simulink model "AutoManualManeuver"  (R2017b)
settings: Solver=FixedStepAuto  StartTime=0.0  StopTime=10.0  FixedStep=0.08  RelTol=1e-3
model workspace (MAT data in the model file):
  ContractValidatorBlocksMap = containers.Map
  ContractValidatorBlocksMap.serialization.keys = {'AutoManualManeuver/Logic/If AUTO/AUTO MANEUVER MODULE/req_s3_3_2_p27_1/validator', 'AutoManualManeuver/Logic/Req_s3_1_2_2_p19_5/validator', 'AutoManualManeuver/Logic/Req_s3_1_2_2_p19_5_part2/validator', 'AutoManualManeuver/Req_s3_1_2_2_p19_5_part1/validator', 'AutoManualManeuver/Req_s3_1_2_2_p19_5_part2/validator', 'AutoManualManeuver/contract/validator'}
  ContractValidatorBlocksMap.serialization.values{1}.block = 'AutoManualManeuver/Logic/If AUTO/AUTO MANEUVER MODULE/req_s3_3_2_p27_1/validator'
  ContractValidatorBlocksMap.serialization.values{1}.assumePorts = 1
  ContractValidatorBlocksMap.serialization.values{1}.guaranteePorts = 2
  ContractValidatorBlocksMap.serialization.values{1}.modeBlocksPorts = 0
  ContractValidatorBlocksMap.serialization.values{1}.portHandles.Inport = [4142.00036621 4143.00036621 4144.00036621]
  ContractValidatorBlocksMap.serialization.values{1}.portHandles.Outport = 4145.00036621
  ContractValidatorBlocksMap.serialization.values{1}.portHandles.Enable = []
  ContractValidatorBlocksMap.serialization.values{1}.portHandles.Trigger = []
  ContractValidatorBlocksMap.serialization.values{1}.portHandles.State = []
  ContractValidatorBlocksMap.serialization.values{1}.portHandles.LConn = []
  ContractValidatorBlocksMap.serialization.values{1}.portHandles.RConn = []
  ContractValidatorBlocksMap.serialization.values{1}.portHandles.Ifaction = []
  ContractValidatorBlocksMap.serialization.values{1}.portHandles.Reset = []
  ContractValidatorBlocksMap.serialization.values{1}.portConnectivity(1).Type = '1'
  ContractValidatorBlocksMap.serialization.values{1}.portConnectivity(1).Position = [365 -95]
  ContractValidatorBlocksMap.serialization.values{1}.portConnectivity(1).SrcBlock = 3623.00036621
  ContractValidatorBlocksMap.serialization.values{1}.portConnectivity(1).SrcPort = 0
  ContractValidatorBlocksMap.serialization.values{1}.portConnectivity(1).DstBlock = []
  ContractValidatorBlocksMap.serialization.values{1}.portConnectivity(1).DstPort = []
  ContractValidatorBlocksMap.serialization.values{1}.portConnectivity(2).Type = '2'
  ContractValidatorBlocksMap.serialization.values{1}.portConnectivity(2).Position = [365 75]
  ContractValidatorBlocksMap.serialization.values{1}.portConnectivity(2).SrcBlock = 3631.00061035
  ContractValidatorBlocksMap.serialization.values{1}.portConnectivity(2).SrcPort = 0
  ContractValidatorBlocksMap.serialization.values{1}.portConnectivity(2).DstBlock = []
  ContractValidatorBlocksMap.serialization.values{1}.portConnectivity(2).DstPort = []
  ContractValidatorBlocksMap.serialization.values{1}.portConnectivity(3).Type = '3'
  ContractValidatorBlocksMap.serialization.values{1}.portConnectivity(3).Position = [365 245]
  ContractValidatorBlocksMap.serialization.values{1}.portConnectivity(3).SrcBlock = 3645.00061035
  ContractValidatorBlocksMap.serialization.values{1}.portConnectivity(3).SrcPort = 0
  ContractValidatorBlocksMap.serialization.values{1}.portConnectivity(3).DstBlock = []
  ContractValidatorBlocksMap.serialization.values{1}.portConnectivity(3).DstPort = []
  ContractValidatorBlocksMap.serialization.values{1}.portConnectivity(4).Type = '1'
  ContractValidatorBlocksMap.serialization.values{1}.portConnectivity(4).Position = [500 75]
  ContractValidatorBlocksMap.serialization.values{1}.portConnectivity(4).SrcBlock = []
  ContractValidatorBlocksMap.serialization.values{1}.portConnectivity(4).SrcPort = []
  ContractValidatorBlocksMap.serialization.values{1}.portConnectivity(4).DstBlock = 3658.00036621
  ContractValidatorBlocksMap.serialization.values{1}.portConnectivity(4).DstPort = 0
  ContractValidatorBlocksMap.serialization.values{2}.block = 'AutoManualManeuver/Logic/Req_s3_1_2_2_p19_5/validator'
  ContractValidatorBlocksMap.serialization.values{2}.assumePorts = 0
  ContractValidatorBlocksMap.serialization.values{2}.guaranteePorts = 1
  ContractValidatorBlocksMap.serialization.values{2}.modeBlocksPorts = 0
  ContractValidatorBlocksMap.serialization.values{2}.portHandles.Inport = 9798.00244141
  ContractValidatorBlocksMap.serialization.values{2}.portHandles.Outport = 9719.00170898
  ContractValidatorBlocksMap.serialization.values{2}.portHandles.Enable = []
  ContractValidatorBlocksMap.serialization.values{2}.portHandles.Trigger = []
  ContractValidatorBlocksMap.serialization.values{2}.portHandles.State = []
  ContractValidatorBlocksMap.serialization.values{2}.portHandles.LConn = []
  ContractValidatorBlocksMap.serialization.values{2}.portHandles.RConn = []
  ContractValidatorBlocksMap.serialization.values{2}.portHandles.Ifaction = []
  ContractValidatorBlocksMap.serialization.values{2}.portHandles.Reset = []
  ContractValidatorBlocksMap.serialization.values{2}.portConnectivity(1).Type = '1'
  ContractValidatorBlocksMap.serialization.values{2}.portConnectivity(1).Position = [365 140]
  ContractValidatorBlocksMap.serialization.values{2}.portConnectivity(1).SrcBlock = 9639.00195312
  ContractValidatorBlocksMap.serialization.values{2}.portConnectivity(1).SrcPort = 0
  ContractValidatorBlocksMap.serialization.values{2}.portConnectivity(1).DstBlock = []
  ContractValidatorBlocksMap.serialization.values{2}.portConnectivity(1).DstPort = []
  ContractValidatorBlocksMap.serialization.values{2}.portConnectivity(2).Type = '1'
  ContractValidatorBlocksMap.serialization.values{2}.portConnectivity(2).Position = [515 140]
  ContractValidatorBlocksMap.serialization.values{2}.portConnectivity(2).SrcBlock = []
  ContractValidatorBlocksMap.serialization.values{2}.portConnectivity(2).SrcPort = []
  ContractValidatorBlocksMap.serialization.values{2}.portConnectivity(2).DstBlock = 9656.00195312
  ContractValidatorBlocksMap.serialization.values{2}.portConnectivity(2).DstPort = 0
  ContractValidatorBlocksMap.serialization.values{3}.block = 'AutoManualManeuver/Logic/Req_s3_1_2_2_p19_5_part2/validator'
  ContractValidatorBlocksMap.serialization.values{3}.assumePorts = 0
  ContractValidatorBlocksMap.serialization.values{3}.guaranteePorts = 1
  ContractValidatorBlocksMap.serialization.values{3}.modeBlocksPorts = 0
  ContractValidatorBlocksMap.serialization.values{3}.portHandles.Inport = 10004.0056152
  ContractValidatorBlocksMap.serialization.values{3}.portHandles.Outport = 10005.0059814
  ContractValidatorBlocksMap.serialization.values{3}.portHandles.Enable = []
  ContractValidatorBlocksMap.serialization.values{3}.portHandles.Trigger = []
  ContractValidatorBlocksMap.serialization.values{3}.portHandles.State = []
  ContractValidatorBlocksMap.serialization.values{3}.portHandles.LConn = []
  ContractValidatorBlocksMap.serialization.values{3}.portHandles.RConn = []
  ContractValidatorBlocksMap.serialization.values{3}.portHandles.Ifaction = []
  ContractValidatorBlocksMap.serialization.values{3}.portHandles.Reset = []
  ContractValidatorBlocksMap.serialization.values{3}.portConnectivity(1).Type = '1'
  ContractValidatorBlocksMap.serialization.values{3}.portConnectivity(1).Position = [360 140]
  ContractValidatorBlocksMap.serialization.values{3}.portConnectivity(1).SrcBlock = 8693.01147461
  ContractValidatorBlocksMap.serialization.values{3}.portConnectivity(1).SrcPort = 0
  ContractValidatorBlocksMap.serialization.values{3}.portConnectivity(1).DstBlock = []
  ContractValidatorBlocksMap.serialization.values{3}.portConnectivity(1).DstPort = []
  ContractValidatorBlocksMap.serialization.values{3}.portConnectivity(2).Type = '1'
  ContractValidatorBlocksMap.serialization.values{3}.portConnectivity(2).Position = [515 140]
  ContractValidatorBlocksMap.serialization.values{3}.portConnectivity(2).SrcBlock = []
  ContractValidatorBlocksMap.serialization.values{3}.portConnectivity(2).SrcPort = []
  ContractValidatorBlocksMap.serialization.values{3}.portConnectivity(2).DstBlock = 8698.01123047
  ContractValidatorBlocksMap.serialization.values{3}.portConnectivity(2).DstPort = 0
  ContractValidatorBlocksMap.serialization.values{4}.block = 'AutoManualManeuver/Req_s3_1_2_2_p19_5_part1/validator'
  ContractValidatorBlocksMap.serialization.values{4}.assumePorts = 0
  ContractValidatorBlocksMap.serialization.values{4}.guaranteePorts = 3
  ContractValidatorBlocksMap.serialization.values{4}.modeBlocksPorts = 0
  ContractValidatorBlocksMap.serialization.values{4}.portHandles.Inport = [4138.00061035 4139.00036621 4140.00036621]
  ContractValidatorBlocksMap.serialization.values{4}.portHandles.Outport = 4141.00036621
  ContractValidatorBlocksMap.serialization.values{4}.portHandles.Enable = []
  ContractValidatorBlocksMap.serialization.values{4}.portHandles.Trigger = []
  ContractValidatorBlocksMap.serialization.values{4}.portHandles.State = []
  ContractValidatorBlocksMap.serialization.values{4}.portHandles.LConn = []
  ContractValidatorBlocksMap.serialization.values{4}.portHandles.RConn = []
  ContractValidatorBlocksMap.serialization.values{4}.portHandles.Ifaction = []
  ContractValidatorBlocksMap.serialization.values{4}.portHandles.Reset = []
  ContractValidatorBlocksMap.serialization.values{4}.portConnectivity(1).Type = '1'
  ContractValidatorBlocksMap.serialization.values{4}.portConnectivity(1).Position = [370 -130]
  ContractValidatorBlocksMap.serialization.values{4}.portConnectivity(1).SrcBlock = 4059.00036621
  ContractValidatorBlocksMap.serialization.values{4}.portConnectivity(1).SrcPort = 0
  ContractValidatorBlocksMap.serialization.values{4}.portConnectivity(1).DstBlock = []
  ContractValidatorBlocksMap.serialization.values{4}.portConnectivity(1).DstPort = []
  ContractValidatorBlocksMap.serialization.values{4}.portConnectivity(2).Type = '2'
  ContractValidatorBlocksMap.serialization.values{4}.portConnectivity(2).Position = [370 40]
  ContractValidatorBlocksMap.serialization.values{4}.portConnectivity(2).SrcBlock = 4063.00061035
  ContractValidatorBlocksMap.serialization.values{4}.portConnectivity(2).SrcPort = 0
  ContractValidatorBlocksMap.serialization.values{4}.portConnectivity(2).DstBlock = []
  ContractValidatorBlocksMap.serialization.values{4}.portConnectivity(2).DstPort = []
  ContractValidatorBlocksMap.serialization.values{4}.portConnectivity(3).Type = '3'
  ContractValidatorBlocksMap.serialization.values{4}.portConnectivity(3).Position = [370 210]
  ContractValidatorBlocksMap.serialization.values{4}.portConnectivity(3).SrcBlock = 4067.00061035
  ContractValidatorBlocksMap.serialization.values{4}.portConnectivity(3).SrcPort = 0
  ContractValidatorBlocksMap.serialization.values{4}.portConnectivity(3).DstBlock = []
  ContractValidatorBlocksMap.serialization.values{4}.portConnectivity(3).DstPort = []
  ContractValidatorBlocksMap.serialization.values{4}.portConnectivity(4).Type = '1'
  ContractValidatorBlocksMap.serialization.values{4}.portConnectivity(4).Position = [520 40]
  ContractValidatorBlocksMap.serialization.values{4}.portConnectivity(4).SrcBlock = []
  ContractValidatorBlocksMap.serialization.values{4}.portConnectivity(4).SrcPort = []
  ContractValidatorBlocksMap.serialization.values{4}.portConnectivity(4).DstBlock = 4072.00036621
  ContractValidatorBlocksMap.serialization.values{4}.portConnectivity(4).DstPort = 0
  ContractValidatorBlocksMap.serialization.values{5}.block = 'AutoManualManeuver/Req_s3_1_2_2_p19_5_part2/validator'
  ContractValidatorBlocksMap.serialization.values{5}.assumePorts = 0
  ContractValidatorBlocksMap.serialization.values{5}.guaranteePorts = 1
  ContractValidatorBlocksMap.serialization.values{5}.modeBlocksPorts = 0
  ContractValidatorBlocksMap.serialization.values{5}.portHandles.Inport = 27036.0012207
  ContractValidatorBlocksMap.serialization.values{5}.portHandles.Outport = 27037.0009766
  ContractValidatorBlocksMap.serialization.values{5}.portHandles.Enable = []
  ContractValidatorBlocksMap.serialization.values{5}.portHandles.Trigger = []
  ContractValidatorBlocksMap.serialization.values{5}.portHandles.State = []
  ContractValidatorBlocksMap.serialization.values{5}.portHandles.LConn = []
  ContractValidatorBlocksMap.serialization.values{5}.portHandles.RConn = []
  ContractValidatorBlocksMap.serialization.values{5}.portHandles.Ifaction = []
  ContractValidatorBlocksMap.serialization.values{5}.portHandles.Reset = []
  ContractValidatorBlocksMap.serialization.values{5}.portConnectivity(1).Type = '1'
  ContractValidatorBlocksMap.serialization.values{5}.portConnectivity(1).Position = [360 140]
  ContractValidatorBlocksMap.serialization.values{5}.portConnectivity(1).SrcBlock = 26634.0003662
  ContractValidatorBlocksMap.serialization.values{5}.portConnectivity(1).SrcPort = 0
  ContractValidatorBlocksMap.serialization.values{5}.portConnectivity(1).DstBlock = []
  ContractValidatorBlocksMap.serialization.values{5}.portConnectivity(1).DstPort = []
  ContractValidatorBlocksMap.serialization.values{5}.portConnectivity(2).Type = '1'
  ContractValidatorBlocksMap.serialization.values{5}.portConnectivity(2).Position = [515 140]
  ContractValidatorBlocksMap.serialization.values{5}.portConnectivity(2).SrcBlock = []
  ContractValidatorBlocksMap.serialization.values{5}.portConnectivity(2).SrcPort = []
  ContractValidatorBlocksMap.serialization.values{5}.portConnectivity(2).DstBlock = 26639.0006104
  ContractValidatorBlocksMap.serialization.values{5}.portConnectivity(2).DstPort = 0
  ContractValidatorBlocksMap.serialization.values{6}.block = 'AutoManualManeuver/contract/validator'
  ContractValidatorBlocksMap.serialization.values{6}.assumePorts = 0
  ContractValidatorBlocksMap.serialization.values{6}.guaranteePorts = 4
  ContractValidatorBlocksMap.serialization.values{6}.modeBlocksPorts = 0
  ContractValidatorBlocksMap.serialization.values{6}.portHandles.Inport = [8429.00061035 8433.00061035 8430.00061035 8428.00061035]
  ContractValidatorBlocksMap.serialization.values{6}.portHandles.Outport = 8423.00085449
  ContractValidatorBlocksMap.serialization.values{6}.portHandles.Enable = []
  ContractValidatorBlocksMap.serialization.values{6}.portHandles.Trigger = []
  ContractValidatorBlocksMap.serialization.values{6}.portHandles.State = []
  ContractValidatorBlocksMap.serialization.values{6}.portHandles.LConn = []
  ContractValidatorBlocksMap.serialization.values{6}.portHandles.RConn = []
  ContractValidatorBlocksMap.serialization.values{6}.portHandles.Ifaction = []
  ContractValidatorBlocksMap.serialization.values{6}.portHandles.Reset = []
  ContractValidatorBlocksMap.serialization.values{6}.portConnectivity(1).Type = '1'
  ContractValidatorBlocksMap.serialization.values{6}.portConnectivity(1).Position = [365 -110]
  ContractValidatorBlocksMap.serialization.values{6}.portConnectivity(1).SrcBlock = -1
  ContractValidatorBlocksMap.serialization.values{6}.portConnectivity(1).SrcPort = []
  ContractValidatorBlocksMap.serialization.values{6}.portConnectivity(1).DstBlock = []
  ContractValidatorBlocksMap.serialization.values{6}.portConnectivity(1).DstPort = []
  ContractValidatorBlocksMap.serialization.values{6}.portConnectivity(2).Type = '2'
  ContractValidatorBlocksMap.serialization.values{6}.portConnectivity(2).Position = [365 15]
  ContractValidatorBlocksMap.serialization.values{6}.portConnectivity(2).SrcBlock = 9285.00170898
  ContractValidatorBlocksMap.serialization.values{6}.portConnectivity(2).SrcPort = 0
  ContractValidatorBlocksMap.serialization.values{6}.portConnectivity(2).DstBlock = []
  ContractValidatorBlocksMap.serialization.values{6}.portConnectivity(2).DstPort = []
  ContractValidatorBlocksMap.serialization.values{6}.portConnectivity(3).Type = '3'
  ContractValidatorBlocksMap.serialization.values{6}.portConnectivity(3).Position = [365 140]
  ContractValidatorBlocksMap.serialization.values{6}.portConnectivity(3).SrcBlock = -1
  ContractValidatorBlocksMap.serialization.values{6}.portConnectivity(3).SrcPort = []
  ContractValidatorBlocksMap.serialization.values{6}.portConnectivity(3).DstBlock = []
  ContractValidatorBlocksMap.serialization.values{6}.portConnectivity(3).DstPort = []
  ContractValidatorBlocksMap.serialization.values{6}.portConnectivity(4).Type = '4'
  ContractValidatorBlocksMap.serialization.values{6}.portConnectivity(4).Position = [365 265]
  ContractValidatorBlocksMap.serialization.values{6}.portConnectivity(4).SrcBlock = -1
  ContractValidatorBlocksMap.serialization.values{6}.portConnectivity(4).SrcPort = []
  ContractValidatorBlocksMap.serialization.values{6}.portConnectivity(4).DstBlock = []
  ContractValidatorBlocksMap.serialization.values{6}.portConnectivity(4).DstPort = []
  ContractValidatorBlocksMap.serialization.values{6}.portConnectivity(5).Type = '1'
  ContractValidatorBlocksMap.serialization.values{6}.portConnectivity(5).Position = [500 80]
  ContractValidatorBlocksMap.serialization.values{6}.portConnectivity(5).SrcBlock = []
  ContractValidatorBlocksMap.serialization.values{6}.portConnectivity(5).SrcPort = []
  ContractValidatorBlocksMap.serialization.values{6}.portConnectivity(5).DstBlock = 8346.00061035
  ContractValidatorBlocksMap.serialization.values{6}.portConnectivity(5).DstPort = 0
  ContractValidatorBlocksMap.serialization.uniformity = 0
  ContractValidatorBlocksMap.serialization.keyType = 'char'
  ContractValidatorBlocksMap.serialization.valueType = 'any'
undefined symbols (not defined in the file or in its folder): contractAfterSimulation, ContractAssumeBlock, contractBeforeSimulation, ContractBlock, ContractGuaranteeBlock, ContractValidatorBlock, saveValidatorParameters
libraries: MATLAB_Function_lib x7, sldvlib x5, simulink x1
settings Model: Creator=hbourbou  LastModifiedBy=hbourbou

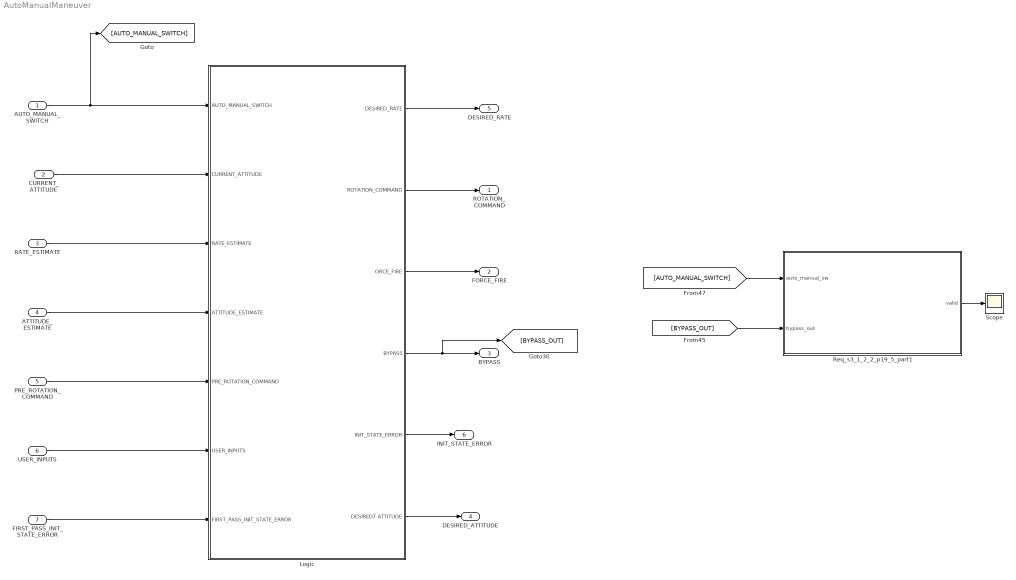
== system AutoManualManeuver ==
  AUTO_MANUAL_SWITCH : Inport  OutDataTypeStr=boolean  PortDimensions=1
  CURRENT_ATTITUDE : Inport  Port=2
  RATE_ESTIMATE : Inport  Port=3
  ATTITUDE_ESTIMATE : Inport  Port=4  PortDimensions=3
  PRE_ROTATION_COMMAND : Inport  Port=5  OutDataTypeStr=double  PortDimensions=3
  USER_INPUTS : Inport  Port=6  OutDataTypeStr=Bus: user_inputsBus
  FIRST_PASS_INIT_STATE_ERROR : Inport  Port=7
  Logic : Subsystem
  Req_s3_1_2_2_p19_5_part1 : Subsystem  mask(ContractBlock){ContractBlockType=ContractBlock}
      mask init:
      | set_param(gcb, 'LinkStatus', 'none');
      settings: CopyFcn=set_param(gcb, 'LinkStatus', 'none');
      mask DialogControl DescTextVar Prompt: Contract block
      mask Display:
      | text(0.5, 0.5, '{\bf\fontsize{20}Contract}', 'hor', 'center', 'texmode','on');
      | blocks = find_system(gcb, 'LookUnderMasks','all', 'SearchDepth',1,'BlockType','Inport');
      | for i = 1 : length(blocks)
      |     blockName = get_param(blocks(i), 'Name');
      |     [path, blockName] = fileparts(char(blockName));
      |     port_label('input', i, blockName);
      | end
      | 
      | blocks = find_system(gcb, 'LookUnderMasks','all', 'SearchDepth',1,'BlockType','Outport');
      | for i = 1 : length(blocks)
      |     blockName = get_param(blocks(i), 'Name');
      |     [path, blockName] = fileparts(char(blockName));
      |     port_label('output', i, blockName);
      | end
  Scope : Scope
  ROTATION_COMMAND : Outport  OutDataTypeStr=double  PortDimensions=3
  FORCE_FIRE : Outport  Port=2
  BYPASS : Outport  Port=3
  DESIRED_ATTITUDE : Outport  Port=4
  DESIRED_RATE : Outport  Port=5  OutDataTypeStr=double
  INIT_STATE_ERROR : Outport  Port=6
  wires:
  [AUTO_MANUAL_SWITCH] -> Req_s3_1_2_2_p19_5_part1/1(auto_manual_sw)
  [BYPASS_OUT] -> Req_s3_1_2_2_p19_5_part1/2(bypass_out)
  Req_s3_1_2_2_p19_5_part1/1(valid) -> Scope/1
  Logic/4(BYPASS) -> [BYPASS_OUT], BYPASS/1
  AUTO_MANUAL_SWITCH/1 -> [AUTO_MANUAL_SWITCH], Logic/1(AUTO_MANUAL_SWITCH)
  CURRENT_ATTITUDE/1 -> Logic/2(CURRENT_ATTITUDE)
  RATE_ESTIMATE/1 -> Logic/3(RATE_ESTIMATE)
  ATTITUDE_ESTIMATE/1 -> Logic/4(ATTITUDE_ESTIMATE)
  PRE_ROTATION_COMMAND/1 -> Logic/5(PRE_ROTATION_COMMAND)
  Logic/1(DESIRED_RATE) -> DESIRED_RATE/1
  Logic/2(ROTATION_COMMAND) -> ROTATION_COMMAND/1
  Logic/3(ORCE_FIRE) -> FORCE_FIRE/1
  USER_INPUTS/1 -> Logic/6(USER_INPUTS)
  FIRST_PASS_INIT_STATE_ERROR/1 -> Logic/7(FIRST_PASS_INIT_STATE_ERROR)
  Logic/6(DESIREDT ATTITUDE) -> DESIRED_ATTITUDE/1
  Logic/5(INIT_STATE_ERROR) -> INIT_STATE_ERROR/1

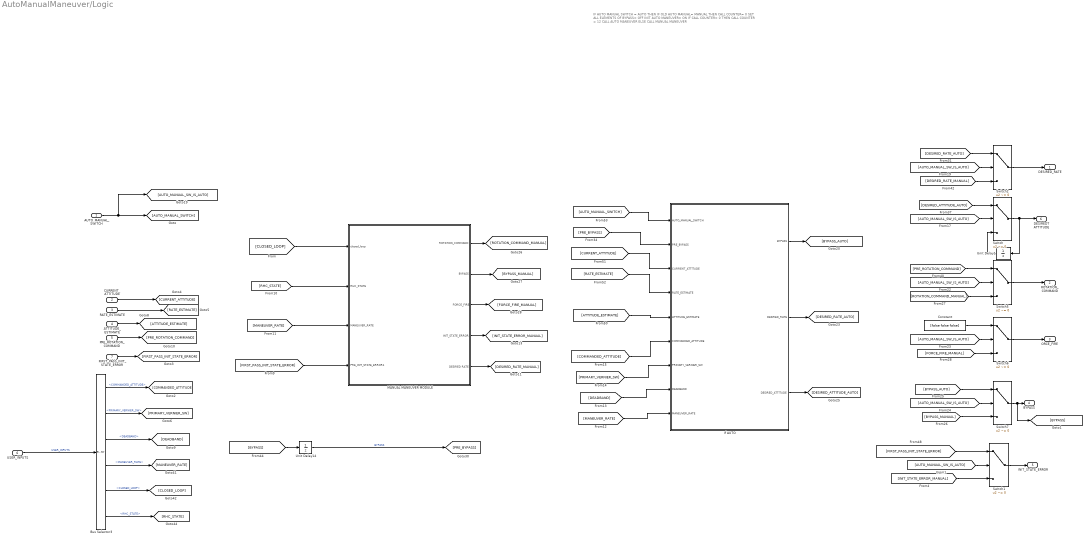
== system AutoManualManeuver/Logic ==
  note: IF AUTO MANUAL SWITCH = AUTO THEN
      | IF OLD AUTO MANUAL= MANUAL THEN
      | CALL COUNTER= 0
      | SET ALL ELEMENTS OF BYPASS= OFF
      | INIT AUTO MANEUVER= ON
      | IF CALL COUNTER= 0 THEN
      | CALL COUNTER = 12
      | CALL AUTO MANEUVER
      | ELSE CALL MANUAL MANEUVER
  AUTO_MANUAL_SWITCH : Inport
  CURRENT_ATTITUDE : Inport  Port=2
  RATE_ESTIMATE : Inport  Port=3
  ATTITUDE_ESTIMATE : Inport  Port=4
  PRE_ROTATION_COMMAND : Inport  Port=5
  USER_INPUTS : Inport  Port=6
  FIRST_PASS_INIT_STATE_ERROR : Inport  Port=7
  Bus Selector3 : BusSelector  OutputSignals=COMMANDED_ATTITUDE,PRIMARY_VERNIER_SW,DEADBAND,MANEUVER_RATE,CLOSED_LOOP,RHC_STATE
  Constant : Constant  Value=[false false false]
  If AUTO : Subsystem  TreatAsAtomicUnit=on
  MANUAL MANEUVER MODULE : Subsystem
  Switch{,1..2,5..7} (6 alike) : Switch  Criteria=u2 ~= 0
  Unit Delay1 : UnitDelay  InitialCondition=[0;0;0]  SampleTime=-1
  Unit Delay14 : UnitDelay  InitialCondition=[true; true; true]  SampleTime=-1
  DESIRED_RATE : Outport  OutDataTypeStr=double
  ROTATION_COMMAND : Outport  Port=2
  ORCE_FIRE : Outport  Port=3
  BYPASS : Outport  Port=4
  INIT_STATE_ERROR : Outport  Port=5
  DESIREDT ATTITUDE : Outport  Port=6  OutDataTypeStr=double
  wires:
  [RHC_STATE] -> MANUAL MANEUVER MODULE/2(RHC_STATE)
  [FIRST_PASS_INIT_STATE_ERROR] -> MANUAL MANEUVER MODULE/4(PRE_INIT_STATE_ERROR1)
  If AUTO/1(BYPASS) -> [BYPASS_AUTO]
  [CLOSED_LOOP] -> MANUAL MANEUVER MODULE/1(closed_loop)
  AUTO_MANUAL_SWITCH/1 -> [AUTO_MANUAL_SWITCH], [AUTO_MANUAL_SW_IS_AUTO]
  PRE_ROTATION_COMMAND/1 -> [PRE_ROTATION_COMMAND]
  [PRE_BYPASS] -> If AUTO/2(PRE_BYPASS)
  [AUTO_MANUAL_SWITCH] -> If AUTO/1(AUTO_MANUAL_SWITCH)
  [CURRENT_ATTITUDE] -> If AUTO/3(CURRENT_ATTITUDE)
  RATE_ESTIMATE/1 -> [RATE_ESTIMATE]
  ATTITUDE_ESTIMATE/1 -> [ATTITUDE_ESTIMATE]
  [RATE_ESTIMATE] -> If AUTO/4(RATE_ESTIMATE)
  CURRENT_ATTITUDE/1 -> [CURRENT_ATTITUDE]
  [ATTITUDE_ESTIMATE] -> If AUTO/5(ATTITUDE_ESTIMATE)
  Switch2/1 -> DESIRED_RATE/1
  Switch7/1 -> [BYPASS], BYPASS/1
  Switch5/1 -> ROTATION_COMMAND/1
  [MANEUVER_RATE] -> If AUTO/9(MANEUVER_RATE)
  [MANEUVER_RATE] -> MANUAL MANEUVER MODULE/3(MANEUVER_RATE)
  [COMMANDED_ATTITUDE] -> If AUTO/6(COMMANDED_ATTITUDE)
  Constant/1 -> Switch6/1
  [DEADBAND] -> If AUTO/8(DEADBAND)
  [PRE_ROTATION_COMMAND] -> Switch5/1
  [PRIMARY_VERNIER_SW] -> If AUTO/7(PRIMARY_VERNIER_SW)
  If AUTO/2(DESIRED_RATE) -> [DESIRED_RATE_AUTO]
  MANUAL MANEUVER MODULE/1(ROTATION_COMMAND) -> [ROTATION_COMMAND_MANUAL]
  MANUAL MANEUVER MODULE/2(BYPASS) -> [BYPASS_MANUAL]
  [DESIRED_RATE_MANUAL] -> Switch2/3
  [AUTO_MANUAL_SW_IS_AUTO] -> Switch2/2
  [DESIRED_RATE_AUTO] -> Switch2/1
  [ROTATION_COMMAND_MANUAL] -> Switch5/3
  [AUTO_MANUAL_SW_IS_AUTO] -> Switch7/2
  [AUTO_MANUAL_SW_IS_AUTO] -> Switch6/2
  [DESIRED_ATTITUDE_AUTO] -> Switch/1
  [BYPASS_MANUAL] -> Switch7/3
  [AUTO_MANUAL_SW_IS_AUTO] -> Switch5/2
  [FORCE_FIRE_MANUAL] -> Switch6/3
  [AUTO_MANUAL_SW_IS_AUTO] -> Switch/2
  If AUTO/3(DESIRED_ATTITUDE) -> [DESIRED_ATTITUDE_AUTO]
  MANUAL MANEUVER MODULE/3(FORCE_FIRE) -> [FORCE_FIRE_MANUAL]
  [BYPASS_AUTO] -> Switch7/1
  [BYPASS] -> Unit Delay14/1
  Unit Delay14/1 -> [PRE_BYPASS]  "BYPASS"
  Switch6/1 -> ORCE_FIRE/1
  Bus Selector3/6 -> [RHC_STATE]  "<RHC_STATE>"
  Bus Selector3/2 -> [PRIMARY_VERNIER_SW]  "<PRIMARY_VERNIER_SW>"
  Bus Selector3/5 -> [CLOSED_LOOP]  "<CLOSED_LOOP>"
  Bus Selector3/1 -> [COMMANDED_ATTITUDE]  "<COMMANDED_ATTITUDE>"
  Bus Selector3/3 -> [DEADBAND]  "<DEADBAND>"
  Bus Selector3/4 -> [MANEUVER_RATE]  "<MANEUVER_RATE>"
  USER_INPUTS/1 -> Bus Selector3/1  "USER_INPUTS"
  FIRST_PASS_INIT_STATE_ERROR/1 -> [FIRST_PASS_INIT_STATE_ERROR]
  MANUAL MANEUVER MODULE/5(DESIRED RATE) -> [DESIRED_RATE_MANUAL]
  [INIT_STATE_ERROR_MANUAL] -> Switch1/3
  [AUTO_MANUAL_SW_IS_AUTO] -> Switch1/2
  [FIRST_PASS_INIT_STATE_ERROR] -> Switch1/1
  Switch1/1 -> INIT_STATE_ERROR/1
  MANUAL MANEUVER MODULE/4(INIT_STATE_ERROR) -> [INIT_STATE_ERROR_MANUAL]
  Switch/1 -> Unit Delay1/1, DESIREDT ATTITUDE/1
  Unit Delay1/1 -> Switch/3

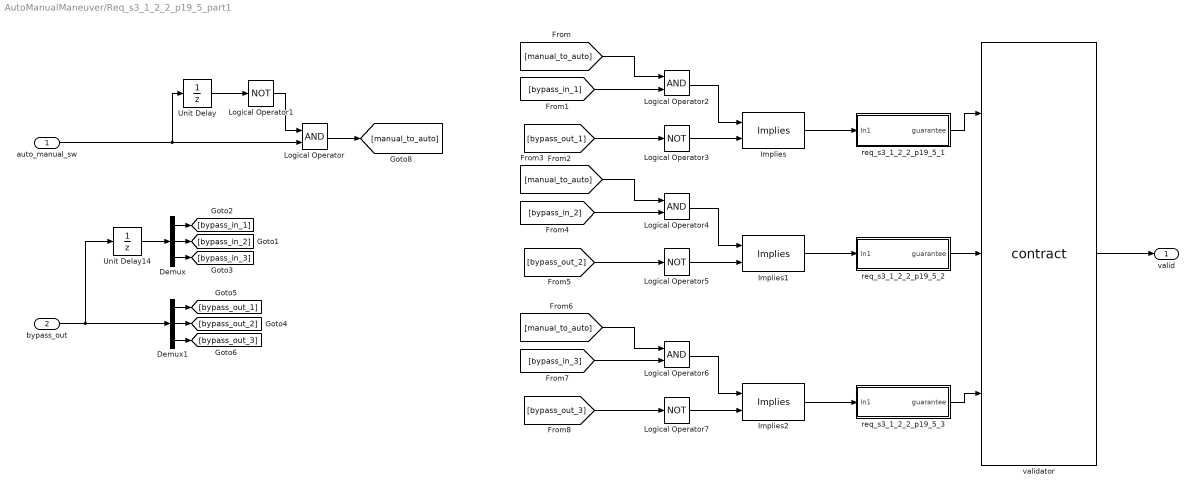
== system AutoManualManeuver/Req_s3_1_2_2_p19_5_part1 ==
  auto_manual_sw : Inport  OutDataTypeStr=boolean  PortDimensions=1
  bypass_out : Inport  Port=2
  Demux : Demux  Outputs=3
  Demux1 : Demux  Outputs=3
  Implies : sldvlib/Verification Utilities/Implies
      settings: SourceProductName=Simulink Design Verifier  SourceProductBaseCode=DV
  Implies1 : sldvlib/Verification Utilities/Implies
      settings: SourceProductName=Simulink Design Verifier  SourceProductBaseCode=DV
  Implies2 : sldvlib/Verification Utilities/Implies
      settings: SourceProductName=Simulink Design Verifier  SourceProductBaseCode=DV
  Logical Operator{,2,4,6} (4 alike) : Logic  AllPortsSameDT=off  OutDataTypeStr=boolean
  Logical Operator1 : Logic  Operator=NOT  Inputs=1  AllPortsSameDT=off  OutDataTypeStr=boolean
  Logical Operator3 : Logic  Operator=NOT  AllPortsSameDT=off  OutDataTypeStr=boolean
  Logical Operator5 : Logic  Operator=NOT  AllPortsSameDT=off  OutDataTypeStr=boolean
  Logical Operator7 : Logic  Operator=NOT  AllPortsSameDT=off  OutDataTypeStr=boolean
  Unit Delay : UnitDelay  InitialCondition=true  SampleTime=-1
  Unit Delay14 : UnitDelay  InitialCondition=[true; true; true]  SampleTime=-1
  req_s3_1_2_2_p19_5_1 : Subsystem  mask(ContractGuaranteeBlock){ContractBlockType=ContractGuaranteeBlock}
      mask init:
      | set_param(gcb, 'LinkStatus', 'none');
      mask DialogControl DescTextVar Prompt: Guarantee block
  req_s3_1_2_2_p19_5_2 : Subsystem  mask(ContractGuaranteeBlock){ContractBlockType=ContractGuaranteeBlock}
      mask init:
      | set_param(gcb, 'LinkStatus', 'none');
      mask DialogControl DescTextVar Prompt: Guarantee block
  req_s3_1_2_2_p19_5_3 : Subsystem  mask(ContractGuaranteeBlock){ContractBlockType=ContractGuaranteeBlock}
      mask init:
      | set_param(gcb, 'LinkStatus', 'none');
      mask DialogControl DescTextVar Prompt: Guarantee block
  validator : M-S-Function  LoadFcn=saveValidatorParameters(gcb);  InitFcn=contractBeforeSimulation();  StopFcn=contractAfterSimulation();  FunctionName=contract  mask(ContractValidatorBlock){assumePorts=0, guaranteePorts=3, modePorts=0, ContractBlockType=ContractValidatorBlock, createInportsCheckbox=off}
      mask prompts: assumePorts "Assume ports     :"; guaranteePorts "Guarantee ports :"; modePorts "Mode ports        :"; createInportsCheckbox "Create inports and connect them automatically"
      mask init:
      | set_param(gcb,'LinkStatus','none');
      | contract_callback('inputs_callback',gcb);
      mask DialogControl DescTextVar Prompt: The validator block implements the following logic: <br> <br> <b>Sofar</b>(assume<sub>1</sub> <b>&#8743;</b> assume<sub>2</sub> <b>&#8743;</b> ... assume<sub>k</sub>) <b>&rarr;</b> (guarantee<sub>1</sub> <b>&#8743;</b> guarantee<sub>2</sub> <b>&#8743;</b> ... guarantee<sub>m</sub> <b>&#8743;</b>  mode<sub>1</sub> <b>&#8743;</b> mode<sub>2</sub> <b>&#8743;</b> ... <b>&#8743;</b> mode<sub>n</sub> )<br> where mode<sub>i</sub> = require<sub>i</sub> <b>&rarr;</b> ensure<sub>i</sub>
      mask Display:
      | color('black');
      | port_label('input',1,'guarantee');
      | port_label('input',2,'guarantee');
      | port_label('input',3,'guarantee');
      | port_label('output',1,'valid');
  valid : Outport
  wires:
  validator/1 -> valid/1
  req_s3_1_2_2_p19_5_3/1(guarantee) -> validator/3
  Implies/1 -> req_s3_1_2_2_p19_5_1/1(In1)
  [manual_to_auto] -> Logical Operator2/1
  Demux/3 -> [bypass_in_3]
  Implies2/1 -> req_s3_1_2_2_p19_5_3/1(In1)
  Logical Operator3/1 -> Implies/2
  [bypass_in_3] -> Logical Operator6/2
  Unit Delay/1 -> Logical Operator1/1
  Demux1/2 -> [bypass_out_2]
  Demux/1 -> [bypass_in_1]
  Logical Operator1/1 -> Logical Operator/1
  bypass_out/1 -> Unit Delay14/1, Demux1/1
  Demux/2 -> [bypass_in_2]
  [bypass_out_1] -> Logical Operator3/1
  [manual_to_auto] -> Logical Operator4/1
  Logical Operator7/1 -> Implies2/2
  Logical Operator2/1 -> Implies/1
  [bypass_out_2] -> Logical Operator5/1
  Implies1/1 -> req_s3_1_2_2_p19_5_2/1(In1)
  [bypass_out_3] -> Logical Operator7/1
  Logical Operator5/1 -> Implies1/2
  [bypass_in_1] -> Logical Operator2/2
  Logical Operator4/1 -> Implies1/1
  Demux1/1 -> [bypass_out_1]
  Unit Delay14/1 -> Demux/1
  [bypass_in_2] -> Logical Operator4/2
  auto_manual_sw/1 -> Logical Operator/2, Unit Delay/1
  Demux1/3 -> [bypass_out_3]
  Logical Operator6/1 -> Implies2/1
  [manual_to_auto] -> Logical Operator6/1
  Logical Operator/1 -> [manual_to_auto]
  req_s3_1_2_2_p19_5_2/1(guarantee) -> validator/2
  req_s3_1_2_2_p19_5_1/1(guarantee) -> validator/1

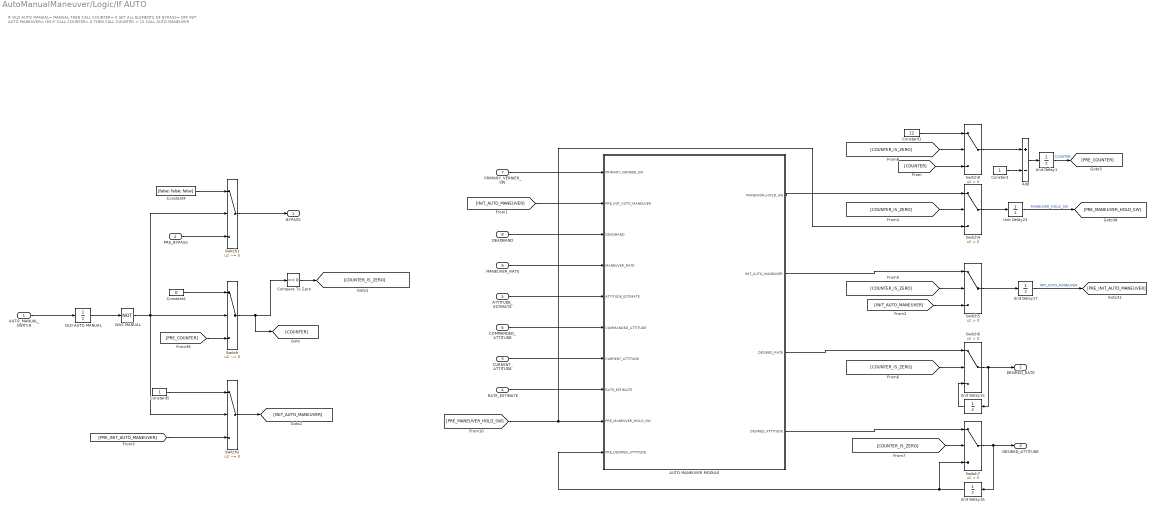
== system AutoManualManeuver/Logic/If AUTO ==
  note: IF OLD AUTO MANUAL= MANUAL THEN
      | CALL COUNTER= 0
      | SET ALL ELEMENTS OF BYPASS= OFF
      | INIT AUTO MANEUVER= ON
      | IF CALL COUNTER= 0 THEN
      | CALL COUNTER = 12
      | CALL AUTO MANEUVER
  AUTO_MANUAL_SWITCH : Inport
  PRE_BYPASS : Inport  Port=2
  CURRENT_ATTITUDE : Inport  Port=3
  RATE_ESTIMATE : Inport  Port=4
  ATTITUDE_ESTIMATE : Inport  Port=5
  COMMANDED_ATTITUDE : Inport  Port=6
  PRIMARY_VERNIER_SW : Inport  Port=7
  DEADBAND : Inport  Port=8
  MANEUVER_RATE : Inport  Port=9
  AUTO MANEUVER MODULE : Subsystem
  Add : Sum  Inputs=+-
  Compare To Zero : simulink/Logic and Bit Operations/Compare To Zero  relop===  OutDataTypeStr=boolean
  Constant : Constant  OutDataTypeStr=uint8  SampleTime=-1
  Constant1 : Constant  Value=12  OutDataTypeStr=uint8
  Constant2 : Constant  Value=0  OutDataTypeStr=uint8
  Constant4 : Constant  Value=[false; false; false]  OutDataTypeStr=boolean
  Constant5 : Constant  OutDataTypeStr=boolean
  OLD AUTO MANUAL : UnitDelay  InitialCondition=false  SampleTime=-1
  Switch : Switch  Criteria=u2 ~= 0
  Switch1 : Switch  Criteria=u2 ~= 0
  Switch2 : Switch  Criteria=u2 ~= 0
  Switch{4..8} (5 alike) : Switch  Criteria=u2 > Threshold
  Unit Delay1 : UnitDelay  SampleTime=-1
  Unit Delay15 : UnitDelay  InitialCondition=[0;0;0]  SampleTime=-1
  Unit Delay16 : UnitDelay  InitialCondition=[0;0;0]  SampleTime=-1
  Unit Delay17 : UnitDelay  InitialCondition=true  SampleTime=-1
  Unit Delay23 : UnitDelay  InitialCondition=[false; false]  SampleTime=-1
  WAS MANUAL : Logic  Operator=NOT  Inputs=1  AllPortsSameDT=off  OutDataTypeStr=boolean
  BYPASS : Outport
  DESIRED_RATE : Outport  Port=2
  DESIRED_ATTITUDE : Outport  Port=3
  wires:
  AUTO_MANUAL_SWITCH/1 -> OLD AUTO MANUAL/1
  Constant2/1 -> Switch/1
  OLD AUTO MANUAL/1 -> WAS MANUAL/1
  Switch1/1 -> BYPASS/1
  Switch5/1 -> Unit Delay17/1
  Constant4/1 -> Switch1/1
  PRE_BYPASS/1 -> Switch1/3
  [PRE_INIT_AUTO_MANEUVER] -> Switch2/3
  Constant5/1 -> Switch2/1
  Constant1/1 -> Switch8/1
  Switch/1 -> [COUNTER], Compare To Zero/1
  AUTO MANEUVER MODULE/2(INIT_AUTO_MANEUVER) -> Switch5/1
  AUTO MANEUVER MODULE/3(DESIRED_RATE) -> Switch6/1
  Switch6/1 -> Unit Delay15/1, DESIRED_RATE/1
  AUTO MANEUVER MODULE/4(DESIRED_ATTITUDE) -> Switch7/1
  AUTO MANEUVER MODULE/1(MANEUVER_HOLD_SW) -> Switch4/1
  MANEUVER_RATE/1 -> AUTO MANEUVER MODULE/4(MANEUVER_RATE)
  DEADBAND/1 -> AUTO MANEUVER MODULE/3(DEADBAND)
  PRIMARY_VERNIER_SW/1 -> AUTO MANEUVER MODULE/1(PRIMARY_VERNIER_SW)
  COMMANDED_ATTITUDE/1 -> AUTO MANEUVER MODULE/6(COMMANDED_ATTITUDE)
  ATTITUDE_ESTIMATE/1 -> AUTO MANEUVER MODULE/5(ATTITUDE_ESTIMATE)
  [PRE_MANEUVER_HOLD_SW] -> AUTO MANEUVER MODULE/9(PRE_MANEUVER_HOLD_SW), Switch4/3
  RATE_ESTIMATE/1 -> AUTO MANEUVER MODULE/8(RATE_ESTIMATE)
  CURRENT_ATTITUDE/1 -> AUTO MANEUVER MODULE/7(CURRENT_ATTITUDE)
  WAS MANUAL/1 -> Switch2/2, Switch1/2, Switch/2
  [COUNTER] -> Switch8/3
  Compare To Zero/1 -> [COUNTER_IS_ZERO]
  [INIT_AUTO_MANEUVER] -> AUTO MANEUVER MODULE/2(PRE_INIT_AUTO_MANEUVER)
  [INIT_AUTO_MANEUVER] -> Switch5/3
  Switch2/1 -> [INIT_AUTO_MANEUVER]
  [COUNTER_IS_ZERO] -> Switch4/2
  [COUNTER_IS_ZERO] -> Switch5/2
  [COUNTER_IS_ZERO] -> Switch6/2
  Unit Delay15/1 -> Switch6/3
  [COUNTER_IS_ZERO] -> Switch7/2
  [COUNTER_IS_ZERO] -> Switch8/2
  Switch8/1 -> Add/1
  Unit Delay1/1 -> [PRE_COUNTER]  "COUNTER"
  [PRE_COUNTER] -> Switch/3
  Unit Delay17/1 -> [PRE_INIT_AUTO_MANEUVER]  "INIT_AUTO_MANEUVER"
  Constant/1 -> Add/2
  Add/1 -> Unit Delay1/1
  Switch7/1 -> Unit Delay16/1, DESIRED_ATTITUDE/1
  Unit Delay16/1 -> Switch7/3, AUTO MANEUVER MODULE/10(PRE_DESIRED_ATTITUDE)
  Switch4/1 -> Unit Delay23/1
  Unit Delay23/1 -> [PRE_MANEUVER_HOLD_SW]  "MANEUVER_HOLD_SW"

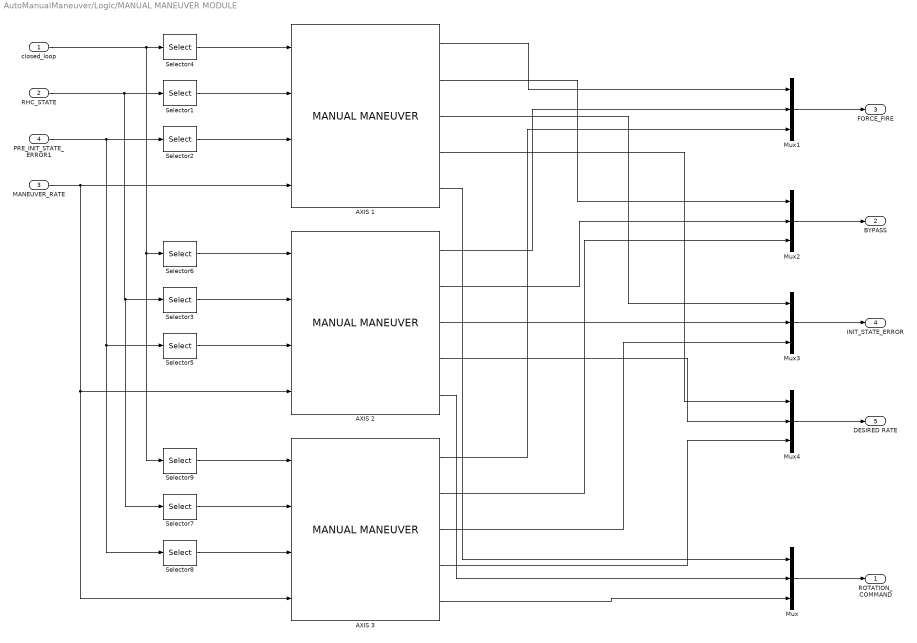
== system AutoManualManeuver/Logic/MANUAL MANEUVER MODULE ==
  closed_loop : Inport
  RHC_STATE : Inport  Port=2
  MANEUVER_RATE : Inport  Port=3
  PRE_INIT_STATE_ERROR1 : Inport  Port=4  OutDataTypeStr=boolean  PortDimensions=3
  AXIS 1 : MATLAB_Function_lib/MANUAL MANEUVER
  AXIS 2 : MATLAB_Function_lib/MANUAL MANEUVER
  AXIS 3 : MATLAB_Function_lib/MANUAL MANEUVER
  Mux{,1..4} (5 alike) : Mux  Inputs=3
  Selector1 : Selector  InputPortWidth=3  IndexOptions=Index vector (dialog)  Indices=1  OutputSizes=1
  Selector2 : Selector  InputPortWidth=3  IndexOptions=Index vector (dialog)  Indices=1  OutputSizes=1
  Selector3 : Selector  InputPortWidth=3  IndexOptions=Index vector (dialog)  Indices=2  OutputSizes=1
  Selector4 : Selector  InputPortWidth=3  IndexOptions=Index vector (dialog)  Indices=1  OutputSizes=1
  Selector5 : Selector  InputPortWidth=3  IndexOptions=Index vector (dialog)  Indices=2  OutputSizes=1
  Selector6 : Selector  InputPortWidth=3  IndexOptions=Index vector (dialog)  Indices=2  OutputSizes=1
  Selector7 : Selector  InputPortWidth=3  IndexOptions=Index vector (dialog)  Indices=3  OutputSizes=1
  Selector8 : Selector  InputPortWidth=3  IndexOptions=Index vector (dialog)  Indices=3  OutputSizes=1
  Selector9 : Selector  InputPortWidth=3  IndexOptions=Index vector (dialog)  Indices=3  OutputSizes=1
  ROTATION_COMMAND : Outport
  BYPASS : Outport  Port=2
  FORCE_FIRE : Outport  Port=3  OutDataTypeStr=boolean  PortDimensions=3
  INIT_STATE_ERROR : Outport  Port=4
  DESIRED RATE : Outport  Port=5
  wires:
  Mux/1 -> ROTATION_COMMAND/1
  Mux2/1 -> BYPASS/1
  Mux1/1 -> FORCE_FIRE/1
  Selector4/1 -> AXIS 1/1
  Selector1/1 -> AXIS 1/2
  Selector2/1 -> AXIS 1/3
  MANEUVER_RATE/1 -> AXIS 2/4, AXIS 3/4, AXIS 1/4
  closed_loop/1 -> Selector9/1, Selector6/1, Selector4/1
  PRE_INIT_STATE_ERROR1/1 -> Selector5/1, Selector8/1, Selector2/1
  Mux3/1 -> INIT_STATE_ERROR/1
  Mux4/1 -> DESIRED RATE/1
  AXIS 1/1 -> Mux1/1
  AXIS 2/1 -> Mux1/2
  AXIS 3/1 -> Mux1/3
  AXIS 1/2 -> Mux2/1
  AXIS 2/2 -> Mux2/2
  AXIS 3/2 -> Mux2/3
  AXIS 1/3 -> Mux3/1
  AXIS 2/3 -> Mux3/2
  AXIS 3/3 -> Mux3/3
  AXIS 1/4 -> Mux4/1
  AXIS 2/4 -> Mux4/2
  AXIS 3/4 -> Mux4/3
  AXIS 3/5 -> Mux/3
  AXIS 2/5 -> Mux/2
  AXIS 1/5 -> Mux/1
  Selector6/1 -> AXIS 2/1
  Selector3/1 -> AXIS 2/2
  Selector5/1 -> AXIS 2/3
  Selector9/1 -> AXIS 3/1
  Selector7/1 -> AXIS 3/2
  Selector8/1 -> AXIS 3/3
  RHC_STATE/1 -> Selector7/1, Selector3/1, Selector1/1

== system AutoManualManeuver/Req_s3_1_2_2_p19_5_part1/req_s3_1_2_2_p19_5_1 ==
  In1 : Inport
  guarantee : Outport  OutDataTypeStr=boolean
  wires:
  In1/1 -> guarantee/1

== system AutoManualManeuver/Req_s3_1_2_2_p19_5_part1/req_s3_1_2_2_p19_5_2 ==
  In1 : Inport
  guarantee : Outport  OutDataTypeStr=boolean
  wires:
  In1/1 -> guarantee/1

== system AutoManualManeuver/Req_s3_1_2_2_p19_5_part1/req_s3_1_2_2_p19_5_3 ==
  In1 : Inport
  guarantee : Outport  OutDataTypeStr=boolean
  wires:
  In1/1 -> guarantee/1

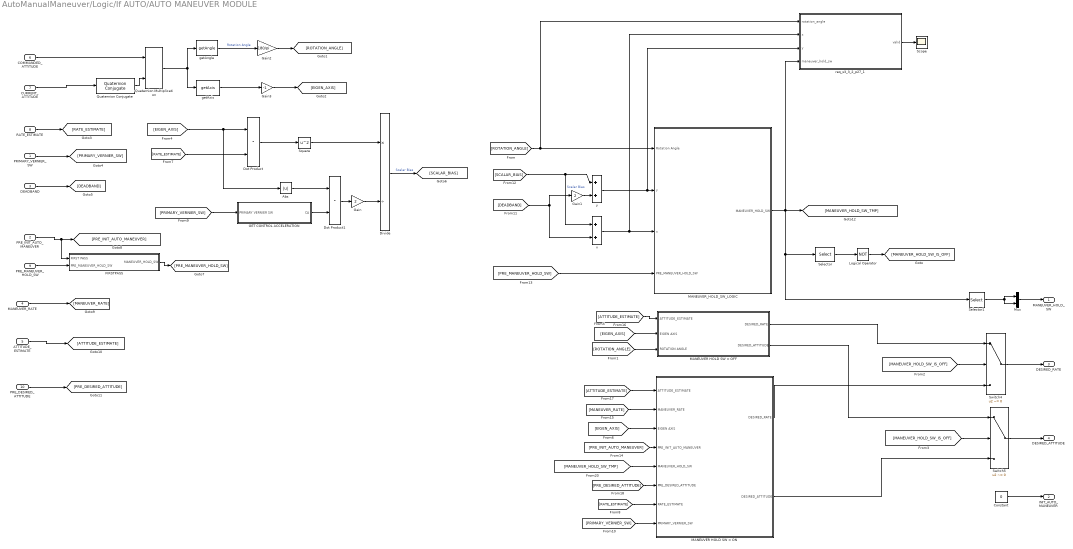
== system AutoManualManeuver/Logic/If AUTO/AUTO MANEUVER MODULE ==
  PRIMARY_VERNIER_SW : Inport
  PRE_INIT_AUTO_MANEUVER : Inport  Port=2
  DEADBAND : Inport  Port=3
  MANEUVER_RATE : Inport  Port=4
  ATTITUDE_ESTIMATE : Inport  Port=5
  COMMANDED_ATTITUDE : Inport  Port=6
  CURRENT_ATTITUDE : Inport  Port=7
  RATE_ESTIMATE : Inport  Port=8
  PRE_MANEUVER_HOLD_SW : Inport  Port=9
  PRE_DESIRED_ATTITUDE : Inport  Port=10
  Abs : Abs
  Constant : Constant  Value=0  OutDataTypeStr=boolean
  Divide : Product  Inputs=*/
  Dot Product : DotProduct  InputSameDT=on  OutDataTypeStr=Inherit: Inherit via internal rule
  Dot Product1 : DotProduct  InputSameDT=on  OutDataTypeStr=Inherit: Inherit via internal rule
  FIRSTPASS : Subsystem
  GET CONTROL ACCELERATION : Subsystem
  Gain : Gain  Gain=2
  Gain1 : Gain  Gain=2
  Gain2 : Gain  Gain=180/pi
  Gain3 : Gain  Gain=-1
  Logical Operator : Logic  Operator=NOT  AllPortsSameDT=off  OutDataTypeStr=boolean
  MANEUVER HOLD SW = OFF : Subsystem  TreatAsAtomicUnit=on
  MANEUVER HOLD SW = ON : Subsystem  TreatAsAtomicUnit=on
  MANEUVER_HOLD_SW_LOGIC : Subsystem
  Mux : Mux  Inputs=2
  Quaternion Conjugate : MATLAB_Function_lib/Quaternion Conjugate
  Quaternion Multiplication : MATLAB_Function_lib/Quaternion Multiplication
  Scope : Scope
  Selector : Selector  InputPortWidth=2  IndexOptions=Index vector (dialog)  Indices=[1]  OutputSizes=1
  Selector1 : Selector  InputPortWidth=2  IndexOptions=Index vector (dialog)  Indices=[1]  OutputSizes=1
  Square : Math  Operator=square  RndMeth=Zero  SaturateOnIntegerOverflow=on
  Switch4 : Switch  Criteria=u2 ~= 0
  Switch5 : Switch  Criteria=u2 ~= 0
  getAngle : MATLAB_Function_lib/getAngle
  getAxis : MATLAB_Function_lib/getAxis
  req_s3_3_2_p27_1 : Subsystem  mask(ContractBlock){ContractBlockType=ContractBlock}
      mask init:
      | set_param(gcb, 'LinkStatus', 'none');
      settings: CopyFcn=set_param(gcb, 'LinkStatus', 'none');
      mask DialogControl DescTextVar Prompt: Contract block
      mask Display:
      | text(0.5, 0.5, '{\bf\fontsize{20}Contract}', 'hor', 'center', 'texmode','on');
      | blocks = find_system(gcb, 'LookUnderMasks','all', 'SearchDepth',1,'BlockType','Inport');
      | for i = 1 : length(blocks)
      |     blockName = get_param(blocks(i), 'Name');
      |     [path, blockName] = fileparts(char(blockName));
      |     port_label('input', i, blockName);
      | end
      | 
      | blocks = find_system(gcb, 'LookUnderMasks','all', 'SearchDepth',1,'BlockType','Outport');
      | for i = 1 : length(blocks)
      |     blockName = get_param(blocks(i), 'Name');
      |     [path, blockName] = fileparts(char(blockName));
      |     port_label('output', i, blockName);
      | end
  x : Sum
  y : Sum
  MANEUVER_HOLD_SW : Outport
  INIT_AUTO_MANEUVER : Outport  Port=2
  DESIRED_RATE : Outport  Port=3
  DESIRED_ATTITUDE : Outport  Port=4
  wires:
  Gain/1 -> Divide/2
  [SCALAR_BIAS] -> x/1, y/1  "Scalar Bias"
  Selector/1 -> Logical Operator/1
  getAxis/1 -> Gain3/1
  Gain1/1 -> y/2
  GET CONTROL ACCELERATION/1(CA) -> Dot Product1/2
  Square/1 -> Divide/1
  Dot Product1/1 -> Gain/1
  getAngle/1 -> Gain2/1  "Rotation Angle"
  Abs/1 -> Dot Product1/1
  Quaternion Multiplication/1 -> getAngle/1, getAxis/1
  Quaternion Conjugate/1 -> Quaternion Multiplication/2
  Dot Product/1 -> Square/1
  [EIGEN_AXIS] -> Dot Product/1, Abs/1
  CURRENT_ATTITUDE/1 -> Quaternion Conjugate/1
  [DEADBAND] -> x/2, Gain1/1
  COMMANDED_ATTITUDE/1 -> Quaternion Multiplication/1
  MANEUVER HOLD SW = OFF/1(DESIRED_RATE) -> Switch4/1
  MANEUVER HOLD SW = ON/1(DESIRED_RATE) -> Switch4/3
  Switch4/1 -> DESIRED_RATE/1
  MANEUVER HOLD SW = ON/2(DESIRED_ATTITUDE) -> Switch5/3
  Switch5/1 -> DESIRED_ATTITUDE/1
  Selector1/1 -> Mux/2, Mux/1
  Logical Operator/1 -> [MANEUVER_HOLD_SW_IS_OFF]
  [MANEUVER_HOLD_SW_IS_OFF] -> Switch4/2
  [MANEUVER_HOLD_SW_IS_OFF] -> Switch5/2
  x/1 -> req_s3_3_2_p27_1/2(x), MANEUVER_HOLD_SW_LOGIC/3(x)
  y/1 -> req_s3_3_2_p27_1/3(y), MANEUVER_HOLD_SW_LOGIC/2(y)
  req_s3_3_2_p27_1/1(valid) -> Scope/1
  [ROTATION_ANGLE] -> req_s3_3_2_p27_1/1(rotation_angle), MANEUVER_HOLD_SW_LOGIC/1(Rotation Angle)
  Mux/1 -> MANEUVER_HOLD_SW/1
  PRE_MANEUVER_HOLD_SW/1 -> FIRSTPASS/2(PRE_MANEUVER_HOLD_SW)
  Constant/1 -> INIT_AUTO_MANEUVER/1
  Gain2/1 -> [ROTATION_ANGLE]
  [ROTATION_ANGLE] -> MANEUVER HOLD SW = OFF/3(ROTATION ANGLE)
  Gain3/1 -> [EIGEN_AXIS]
  [EIGEN_AXIS] -> MANEUVER HOLD SW = OFF/2(EIGEN AXIS)
  [EIGEN_AXIS] -> MANEUVER HOLD SW = ON/3(EIGEN AXIS)
  RATE_ESTIMATE/1 -> [RATE_ESTIMATE]
  [RATE_ESTIMATE] -> Dot Product/2
  [RATE_ESTIMATE] -> MANEUVER HOLD SW = ON/7(RATE_ESTIMATE)
  PRIMARY_VERNIER_SW/1 -> [PRIMARY_VERNIER_SW]
  [PRIMARY_VERNIER_SW] -> GET CONTROL ACCELERATION/1(PRIMARY VERNIER SW)
  [PRIMARY_VERNIER_SW] -> MANEUVER HOLD SW = ON/8(PRIMARY_VERNIER_SW)
  DEADBAND/1 -> [DEADBAND]
  Divide/1 -> [SCALAR_BIAS]  "Scalar Bias"
  FIRSTPASS/1(MANEUVER_HOLD_SW) -> [PRE_MANEUVER_HOLD_SW]
  [PRE_MANEUVER_HOLD_SW] -> MANEUVER_HOLD_SW_LOGIC/4(PRE_MANEUVER_HOLD_SW)
  PRE_INIT_AUTO_MANEUVER/1 -> FIRSTPASS/1(FIRST PASS), [PRE_INIT_AUTO_MANEUVER]
  [PRE_INIT_AUTO_MANEUVER] -> MANEUVER HOLD SW = ON/4(PRE_INIT_AUTO_MANEUVER)
  MANEUVER_RATE/1 -> [MANEUVER_RATE]
  [MANEUVER_RATE] -> MANEUVER HOLD SW = ON/2(MANEUVER_RATE)
  ATTITUDE_ESTIMATE/1 -> [ATTITUDE_ESTIMATE]
  [ATTITUDE_ESTIMATE] -> MANEUVER HOLD SW = OFF/1(ATTITUDE_ESTIMATE)
  [ATTITUDE_ESTIMATE] -> MANEUVER HOLD SW = ON/1(ATTITUDE_ESTIMATE)
  PRE_DESIRED_ATTITUDE/1 -> [PRE_DESIRED_ATTITUDE]
  [PRE_DESIRED_ATTITUDE] -> MANEUVER HOLD SW = ON/6(PRE_DESIRED_ATTITUDE)
  MANEUVER_HOLD_SW_LOGIC/1(MANEUVER_HOLD_SW) -> req_s3_3_2_p27_1/4(maneuver_hold_sw), Selector1/1, Selector/1, [MANEUVER_HOLD_SW_TMP]
  [MANEUVER_HOLD_SW_TMP] -> MANEUVER HOLD SW = ON/5(MANEUVER_HOLD_SW)
  MANEUVER HOLD SW = OFF/2(DESIRED_ATTITUDE) -> Switch5/1

== system AutoManualManeuver/Logic/If AUTO/AUTO MANEUVER MODULE/FIRSTPASS ==
  note: IF FIRST PASS THEN
      | MANEUVER HOLD SWITCH = OFF
      | OLD MANEUVER HOLD SWITCH = OFF
  FIRST PASS : Inport
  PRE_MANEUVER_HOLD_SW : Inport  Port=2
  Constant : Constant  Value=false
  Mux : Mux  Inputs=2
  Switch : Switch  Criteria=u2 ~= 0
  MANEUVER_HOLD_SW : Outport
  wires:
  Switch/1 -> MANEUVER_HOLD_SW/1
  FIRST PASS/1 -> Switch/2
  PRE_MANEUVER_HOLD_SW/1 -> Switch/3
  Constant/1 -> Mux/2, Mux/1
  Mux/1 -> Switch/1

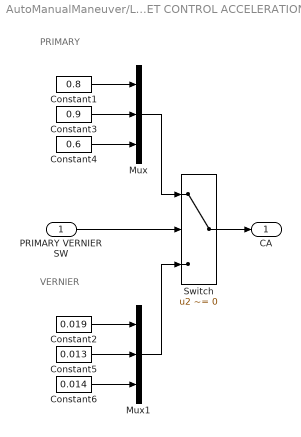
== system AutoManualManeuver/Logic/If AUTO/AUTO MANEUVER MODULE/GET CONTROL ACCELERATION ==
  note: VERNIER
  note: PRIMARY
  PRIMARY VERNIER SW : Inport
  Constant1 : Constant  Value=0.8
  Constant2 : Constant  Value=0.019
  Constant3 : Constant  Value=0.9
  Constant4 : Constant  Value=0.6
  Constant5 : Constant  Value=0.013
  Constant6 : Constant  Value=0.014
  Mux : Mux  Inputs=3
  Mux1 : Mux  Inputs=3
  Switch : Switch  Criteria=u2 ~= 0
  CA : Outport
  wires:
  PRIMARY VERNIER SW/1 -> Switch/2
  Mux/1 -> Switch/1
  Mux1/1 -> Switch/3
  Switch/1 -> CA/1
  Constant4/1 -> Mux/3
  Constant3/1 -> Mux/2
  Constant1/1 -> Mux/1
  Constant2/1 -> Mux1/1
  Constant5/1 -> Mux1/2
  Constant6/1 -> Mux1/3

== system AutoManualManeuver/Logic/If AUTO/AUTO MANEUVER MODULE/MANEUVER HOLD SW = OFF ==
  ATTITUDE_ESTIMATE : Inport
  EIGEN AXIS : Inport  Port=2
  ROTATION ANGLE : Inport  Port=3
  Add : Sum
  Constant : Constant  Value=[0;0;0]
  Product : Product
  DESIRED_RATE : Outport
  DESIRED_ATTITUDE : Outport  Port=2
  wires:
  Constant/1 -> DESIRED_RATE/1
  Add/1 -> DESIRED_ATTITUDE/1
  ROTATION ANGLE/1 -> Product/2
  ATTITUDE_ESTIMATE/1 -> Add/1
  EIGEN AXIS/1 -> Product/1
  Product/1 -> Add/2

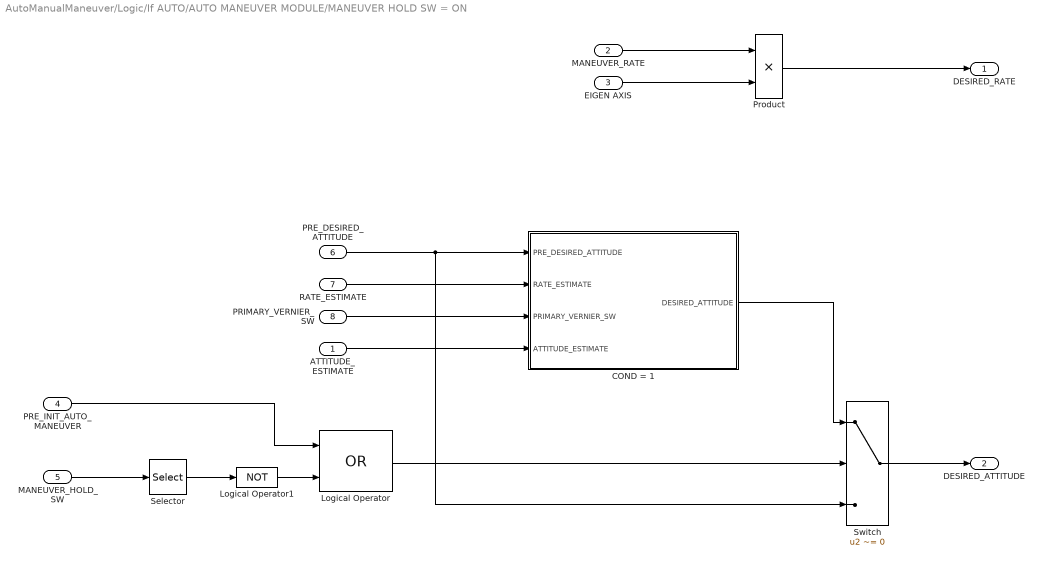
== system AutoManualManeuver/Logic/If AUTO/AUTO MANEUVER MODULE/MANEUVER HOLD SW = ON ==
  ATTITUDE_ESTIMATE : Inport
  MANEUVER_RATE : Inport  Port=2
  EIGEN AXIS : Inport  Port=3
  PRE_INIT_AUTO_MANEUVER : Inport  Port=4
  MANEUVER_HOLD_SW : Inport  Port=5
  PRE_DESIRED_ATTITUDE : Inport  Port=6
  RATE_ESTIMATE : Inport  Port=7
  PRIMARY_VERNIER_SW : Inport  Port=8
  COND = 1 : Subsystem  TreatAsAtomicUnit=on
  Logical Operator : Logic  Operator=OR  AllPortsSameDT=off  OutDataTypeStr=boolean
  Logical Operator1 : Logic  Operator=NOT  AllPortsSameDT=off  OutDataTypeStr=boolean
  Product : Product
  Selector : Selector  InputPortWidth=2  IndexOptions=Index vector (dialog)  Indices=[2]  OutputSizes=1
  Switch : Switch  Criteria=u2 ~= 0
  DESIRED_RATE : Outport
  DESIRED_ATTITUDE : Outport  Port=2
  wires:
  MANEUVER_RATE/1 -> Product/1
  EIGEN AXIS/1 -> Product/2
  Product/1 -> DESIRED_RATE/1
  Selector/1 -> Logical Operator1/1
  MANEUVER_HOLD_SW/1 -> Selector/1
  PRE_INIT_AUTO_MANEUVER/1 -> Logical Operator/1
  Logical Operator1/1 -> Logical Operator/2
  PRE_DESIRED_ATTITUDE/1 -> COND = 1/1(PRE_DESIRED_ATTITUDE), Switch/3
  COND = 1/1(DESIRED_ATTITUDE) -> Switch/1
  Switch/1 -> DESIRED_ATTITUDE/1
  RATE_ESTIMATE/1 -> COND = 1/2(RATE_ESTIMATE)
  PRIMARY_VERNIER_SW/1 -> COND = 1/3(PRIMARY_VERNIER_SW)
  ATTITUDE_ESTIMATE/1 -> COND = 1/4(ATTITUDE_ESTIMATE)
  Logical Operator/1 -> Switch/2

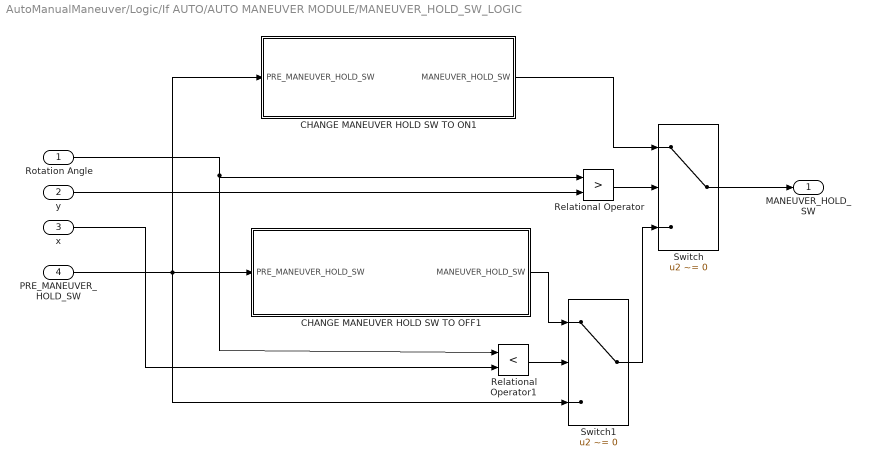
== system AutoManualManeuver/Logic/If AUTO/AUTO MANEUVER MODULE/MANEUVER_HOLD_SW_LOGIC ==
  Rotation Angle : Inport
  y : Inport  Port=2
  x : Inport  Port=3
  PRE_MANEUVER_HOLD_SW : Inport  Port=4
  CHANGE MANEUVER HOLD SW TO OFF1 : Subsystem  TreatAsAtomicUnit=on
  CHANGE MANEUVER HOLD SW TO ON1 : Subsystem  TreatAsAtomicUnit=on
  Relational Operator : RelationalOperator  Operator=>  OutDataTypeStr=boolean  RndMeth=Simplest
  Relational Operator1 : RelationalOperator  Operator=<  OutDataTypeStr=boolean  RndMeth=Simplest
  Switch : Switch  Criteria=u2 ~= 0
  Switch1 : Switch  Criteria=u2 ~= 0
  MANEUVER_HOLD_SW : Outport
  wires:
  Rotation Angle/1 -> Relational Operator1/1, Relational Operator/1
  y/1 -> Relational Operator/2
  x/1 -> Relational Operator1/2
  Switch/1 -> MANEUVER_HOLD_SW/1
  PRE_MANEUVER_HOLD_SW/1 -> CHANGE MANEUVER HOLD SW TO OFF1/1(PRE_MANEUVER_HOLD_SW), Switch1/3, CHANGE MANEUVER HOLD SW TO ON1/1(PRE_MANEUVER_HOLD_SW)
  Relational Operator/1 -> Switch/2
  CHANGE MANEUVER HOLD SW TO ON1/1(MANEUVER_HOLD_SW) -> Switch/1
  Switch1/1 -> Switch/3
  Relational Operator1/1 -> Switch1/2
  CHANGE MANEUVER HOLD SW TO OFF1/1(MANEUVER_HOLD_SW) -> Switch1/1

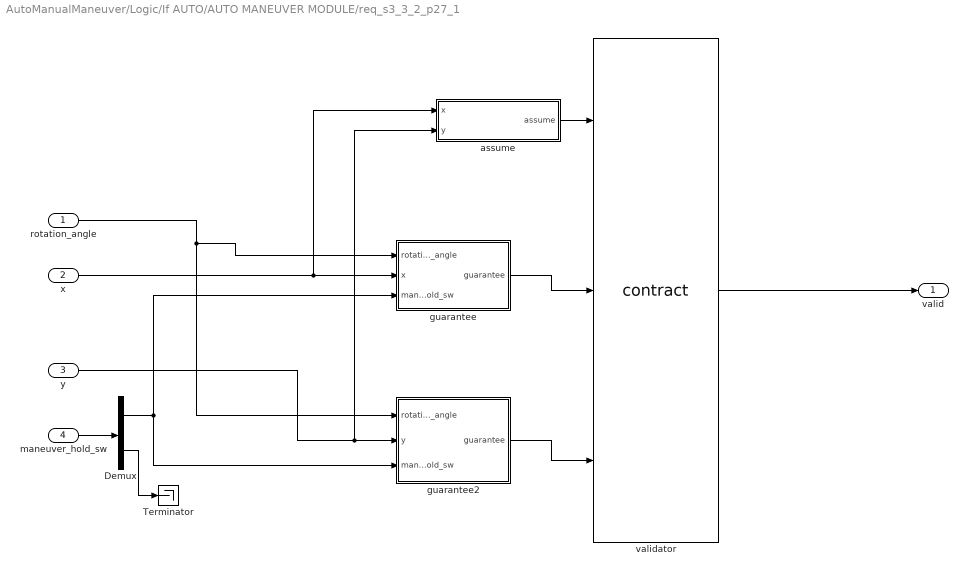
== system AutoManualManeuver/Logic/If AUTO/AUTO MANEUVER MODULE/req_s3_3_2_p27_1 ==
  rotation_angle : Inport
  x : Inport  Port=2
  y : Inport  Port=3
  maneuver_hold_sw : Inport  Port=4  OutDataTypeStr=boolean
  Demux : Demux  Outputs=2
  Terminator : Terminator
  assume : Subsystem  mask(ContractAssumeBlock){ContractBlockType=ContractAssumeBlock}
      mask init:
      | set_param(gcb, 'LinkStatus', 'none');
      mask DialogControl DescTextVar Prompt: Assume block
  guarantee : Subsystem  mask(ContractGuaranteeBlock){ContractBlockType=ContractGuaranteeBlock}
      mask init:
      | set_param(gcb, 'LinkStatus', 'none');
      mask DialogControl DescTextVar Prompt: Guarantee block
  guarantee2 : Subsystem  mask(ContractGuaranteeBlock){ContractBlockType=ContractGuaranteeBlock}
      mask init:
      | set_param(gcb, 'LinkStatus', 'none');
      mask DialogControl DescTextVar Prompt: Guarantee block
  validator : M-S-Function  LoadFcn=saveValidatorParameters(gcb);  InitFcn=contractBeforeSimulation();  StopFcn=contractAfterSimulation();  FunctionName=contract  mask(ContractValidatorBlock){assumePorts=1, guaranteePorts=2, modePorts=0, ContractBlockType=ContractValidatorBlock, createInportsCheckbox=off}
      mask prompts: assumePorts "Assume ports     :"; guaranteePorts "Guarantee ports :"; modePorts "Mode ports        :"; createInportsCheckbox "Create inports and connect them automatically"
      mask init:
      | set_param(gcb,'LinkStatus','none');
      | contract_callback('inputs_callback',gcb);
      mask DialogControl DescTextVar Prompt: The validator block implements the following logic: <br> <br> <b>Sofar</b>(assume<sub>1</sub> <b>&#8743;</b> assume<sub>2</sub> <b>&#8743;</b> ... assume<sub>k</sub>) <b>&rarr;</b> (guarantee<sub>1</sub> <b>&#8743;</b> guarantee<sub>2</sub> <b>&#8743;</b> ... guarantee<sub>m</sub> <b>&#8743;</b>  mode<sub>1</sub> <b>&#8743;</b> mode<sub>2</sub> <b>&#8743;</b> ... <b>&#8743;</b> mode<sub>n</sub> )<br> where mode<sub>i</sub> = require<sub>i</sub> <b>&rarr;</b> ensure<sub>i</sub>
      mask Display:
      | color('black');
      | port_label('input',1,'assume');
      | port_label('input',2,'guarantee');
      | port_label('input',3,'guarantee');
      | port_label('output',1,'valid');
  valid : Outport
  wires:
  x/1 -> assume/1(x), guarantee/2(x)
  rotation_angle/1 -> guarantee/1(rotation_angle), guarantee2/1(rotation_angle)
  validator/1 -> valid/1
  Demux/1 -> guarantee/3(maneuver_hold_sw), guarantee2/3(maneuver_hold_sw)
  y/1 -> assume/2(y), guarantee2/2(y)
  maneuver_hold_sw/1 -> Demux/1
  Demux/2 -> Terminator/1
  guarantee/1(guarantee) -> validator/2
  guarantee2/1(guarantee) -> validator/3
  assume/1(assume) -> validator/1

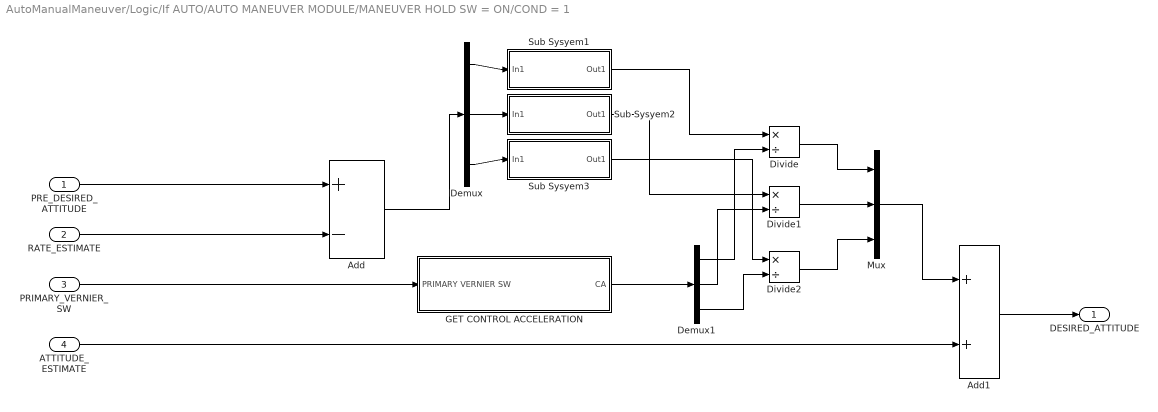
== system AutoManualManeuver/Logic/If AUTO/AUTO MANEUVER MODULE/MANEUVER HOLD SW = ON/COND = 1 ==
  PRE_DESIRED_ATTITUDE : Inport
  RATE_ESTIMATE : Inport  Port=2
  PRIMARY_VERNIER_SW : Inport  Port=3
  ATTITUDE_ESTIMATE : Inport  Port=4
  Add : Sum  Inputs=+-
  Add1 : Sum
  Demux : Demux  Outputs=3
  Demux1 : Demux  Outputs=3
  Divide : Product  Inputs=*/
  Divide1 : Product  Inputs=*/
  Divide2 : Product  Inputs=*/
  GET CONTROL ACCELERATION : Subsystem
  Mux : Mux  Inputs=3
  Sub Sysyem1 : Subsystem
  Sub Sysyem2 : Subsystem
  Sub Sysyem3 : Subsystem
  DESIRED_ATTITUDE : Outport
  wires:
  PRE_DESIRED_ATTITUDE/1 -> Add/1
  RATE_ESTIMATE/1 -> Add/2
  Add/1 -> Demux/1
  PRIMARY_VERNIER_SW/1 -> GET CONTROL ACCELERATION/1(PRIMARY VERNIER SW)
  GET CONTROL ACCELERATION/1(CA) -> Demux1/1
  Demux/1 -> Sub Sysyem1/1(In1)
  Demux/2 -> Sub Sysyem2/1(In1)
  Demux/3 -> Sub Sysyem3/1(In1)
  Sub Sysyem1/1(Out1) -> Divide/1
  Demux1/1 -> Divide/2
  Sub Sysyem2/1(Out1) -> Divide1/1
  Demux1/2 -> Divide1/2
  Sub Sysyem3/1(Out1) -> Divide2/1
  Demux1/3 -> Divide2/2
  Divide/1 -> Mux/1
  Divide1/1 -> Mux/2
  Divide2/1 -> Mux/3
  Mux/1 -> Add1/1
  ATTITUDE_ESTIMATE/1 -> Add1/2
  Add1/1 -> DESIRED_ATTITUDE/1

== system AutoManualManeuver/Logic/If AUTO/AUTO MANEUVER MODULE/MANEUVER_HOLD_SW_LOGIC/CHANGE MANEUVER HOLD SW TO OFF1 ==
  PRE_MANEUVER_HOLD_SW : Inport
  Constant : Constant  Value=0  OutDataTypeStr=boolean
  Demux : Demux  Outputs=2
  Mux : Mux  Inputs=2
  Terminator : Terminator
  MANEUVER_HOLD_SW : Outport
  wires:
  Constant/1 -> Mux/1
  Mux/1 -> MANEUVER_HOLD_SW/1
  PRE_MANEUVER_HOLD_SW/1 -> Demux/1
  Demux/1 -> Terminator/1
  Demux/2 -> Mux/2

== system AutoManualManeuver/Logic/If AUTO/AUTO MANEUVER MODULE/MANEUVER_HOLD_SW_LOGIC/CHANGE MANEUVER HOLD SW TO ON1 ==
  PRE_MANEUVER_HOLD_SW : Inport
  Constant : Constant  OutDataTypeStr=boolean
  Demux : Demux  Outputs=2
  Mux : Mux  Inputs=2
  Terminator : Terminator
  MANEUVER_HOLD_SW : Outport
  wires:
  Mux/1 -> MANEUVER_HOLD_SW/1
  Constant/1 -> Mux/1
  PRE_MANEUVER_HOLD_SW/1 -> Demux/1
  Demux/2 -> Mux/2
  Demux/1 -> Terminator/1

== system AutoManualManeuver/Logic/If AUTO/AUTO MANEUVER MODULE/req_s3_3_2_p27_1/assume ==
  x : Inport
  y : Inport  Port=2
  Relational Operator : RelationalOperator  Operator=>  OutDataTypeStr=boolean  RndMeth=Simplest
  assume : Outport  OutDataTypeStr=boolean
  wires:
  y/1 -> Relational Operator/1
  x/1 -> Relational Operator/2
  Relational Operator/1 -> assume/1

== system AutoManualManeuver/Logic/If AUTO/AUTO MANEUVER MODULE/req_s3_3_2_p27_1/guarantee ==
  rotation_angle : Inport
  x : Inport  Port=2
  maneuver_hold_sw : Inport  Port=3
  Implies : sldvlib/Verification Utilities/Implies
      settings: SourceProductName=Simulink Design Verifier  SourceProductBaseCode=DV
  Logical Operator1 : Logic  Operator=NOT  AllPortsSameDT=off  OutDataTypeStr=boolean
  Relational Operator : RelationalOperator  Operator=<  OutDataTypeStr=boolean  RndMeth=Simplest
  guarantee : Outport  OutDataTypeStr=boolean
  wires:
  Relational Operator/1 -> Implies/1
  Implies/1 -> guarantee/1
  rotation_angle/1 -> Relational Operator/1
  x/1 -> Relational Operator/2
  maneuver_hold_sw/1 -> Logical Operator1/1
  Logical Operator1/1 -> Implies/2

== system AutoManualManeuver/Logic/If AUTO/AUTO MANEUVER MODULE/req_s3_3_2_p27_1/guarantee2 ==
  rotation_angle : Inport
  y : Inport  Port=2
  maneuver_hold_sw : Inport  Port=3
  Implies : sldvlib/Verification Utilities/Implies
      settings: SourceProductName=Simulink Design Verifier  SourceProductBaseCode=DV
  Relational Operator : RelationalOperator  Operator=>  OutDataTypeStr=boolean  RndMeth=Simplest
  guarantee : Outport  OutDataTypeStr=boolean
  wires:
  rotation_angle/1 -> Relational Operator/1
  y/1 -> Relational Operator/2
  Implies/1 -> guarantee/1
  Relational Operator/1 -> Implies/1
  maneuver_hold_sw/1 -> Implies/2

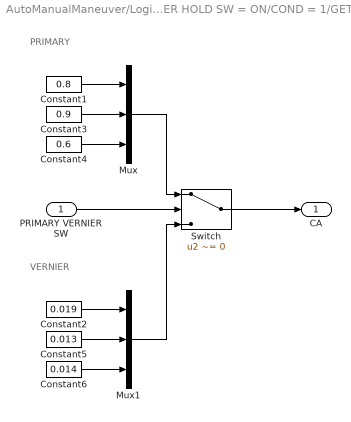
== system AutoManualManeuver/Logic/If AUTO/AUTO MANEUVER MODULE/MANEUVER HOLD SW = ON/COND = 1/GET CONTROL ACCELERATION ==
  note: VERNIER
  note: PRIMARY
  PRIMARY VERNIER SW : Inport
  Constant1 : Constant  Value=0.8
  Constant2 : Constant  Value=0.019
  Constant3 : Constant  Value=0.9
  Constant4 : Constant  Value=0.6
  Constant5 : Constant  Value=0.013
  Constant6 : Constant  Value=0.014
  Mux : Mux  Inputs=3
  Mux1 : Mux  Inputs=3
  Switch : Switch  Criteria=u2 ~= 0
  CA : Outport
  wires:
  PRIMARY VERNIER SW/1 -> Switch/2
  Mux/1 -> Switch/1
  Mux1/1 -> Switch/3
  Switch/1 -> CA/1
  Constant4/1 -> Mux/3
  Constant3/1 -> Mux/2
  Constant1/1 -> Mux/1
  Constant2/1 -> Mux1/1
  Constant5/1 -> Mux1/2
  Constant6/1 -> Mux1/3

== system AutoManualManeuver/Logic/If AUTO/AUTO MANEUVER MODULE/MANEUVER HOLD SW = ON/COND = 1/Sub Sysyem1 ==
  In1 : Inport
  Abs : Abs
  Gain : Gain  Gain=-1
  Product : Product
  Out1 : Outport
  wires:
  Product/1 -> Gain/1
  In1/1 -> Product/1, Abs/1
  Abs/1 -> Product/2
  Gain/1 -> Out1/1

== system AutoManualManeuver/Logic/If AUTO/AUTO MANEUVER MODULE/MANEUVER HOLD SW = ON/COND = 1/Sub Sysyem2 ==
  In1 : Inport
  Abs : Abs
  Gain : Gain  Gain=-1
  Product : Product
  Out1 : Outport
  wires:
  Product/1 -> Gain/1
  In1/1 -> Product/1, Abs/1
  Abs/1 -> Product/2
  Gain/1 -> Out1/1

== system AutoManualManeuver/Logic/If AUTO/AUTO MANEUVER MODULE/MANEUVER HOLD SW = ON/COND = 1/Sub Sysyem3 ==
  In1 : Inport
  Abs : Abs
  Gain : Gain  Gain=-1
  Product : Product
  Out1 : Outport
  wires:
  Product/1 -> Gain/1
  In1/1 -> Product/1, Abs/1
  Abs/1 -> Product/2
  Gain/1 -> Out1/1
